simulink model "my_own_target"  (R2022a)
settings: Solver=VariableStepAuto  StartTime=0.0  StopTime=10.0  RelTol=1e-3
PreLoadFcn:
  | my_own_target_dat
values from neighbouring files (symbols this model uses):
  pos_tgt = [4500+x_ini -h_ini-500]    [my_own_target_dat.m]
  theta_tgt = 180*d2r    (= 3.14159265359)    [my_own_target_dat.m]
  v_tgt = 328    [my_own_target_dat.m]
settings Model: Creator=amani  LastModifiedBy=amani

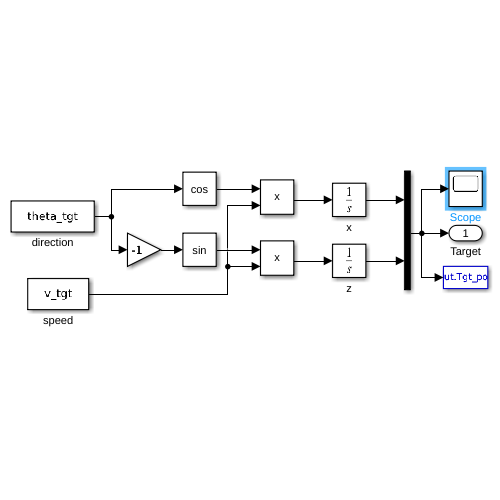
[thumbnail: Simulink's stored preview of the top-level diagram]
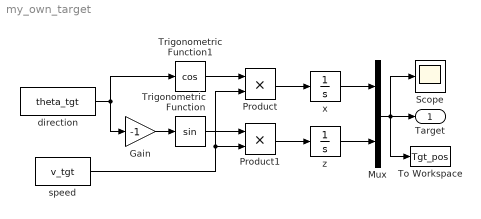
== system my_own_target ==
  Gain : Gain  Gain=-1  SaturateOnIntegerOverflow=on  OutDataTypeStr=Inherit: Same as input  ParamDataTypeStr=Inherit: Same as input
  Mux : Mux  Inputs=2
  Product : Product  InputSameDT=on  SaturateOnIntegerOverflow=on  OutDataTypeStr=Inherit: Same as first input
  Product1 : Product  InputSameDT=on  SaturateOnIntegerOverflow=on  OutDataTypeStr=Inherit: Same as first input
  Scope : Scope
  To Workspace : ToWorkspace  VariableName=Tgt_pos  SaveFormat=Structure  SampleTime=-1
  Trigonometric Function : Trigonometry
  Trigonometric Function1 : Trigonometry  Operator=cos
  direction : Constant  Value=theta_tgt
  speed : Constant  Value=v_tgt
  x : Integrator  InitialCondition=pos_tgt(1)
  z : Integrator  InitialCondition=pos_tgt(2)
  Target : Outport  VectorParamsAs1DForOutWhenUnconnected=off
  wires:
  Gain/1 -> Trigonometric Function/1
  x/1 -> Mux/1
  Product1/1 -> z/1
  speed/1 -> Product/2, Product1/2
  Mux/1 -> Target/1, Scope/1, To Workspace/1
  Trigonometric Function1/1 -> Product/1
  direction/1 -> Trigonometric Function1/1, Gain/1
  Trigonometric Function/1 -> Product1/1
  z/1 -> Mux/2
  Product/1 -> x/1
